simulink model "solid_ofc"  (R2020a)
settings: Solver=VariableStepAuto  StartTime=0.0  StopTime=simulation.stopTime  RelTol=1e-3
values from neighbouring files (symbols this model uses):
  MaxCrossings = 3    [solid_ofc_detection.m]
  Threshold = 0.1    [solid_ofc_detection.m]
  tp = 1/2/pi    (= 0.159154943092)    [solid_ofc_detection.m]
undefined symbols (not defined in the file or in its folder): simulation
libraries: simulink x1, dspsigops x1
settings Model: Creator=FawadFarooq  LastModifiedBy=FawaD KhaN
settings DebuggingCC: SFMachineParentedDataDiag=error

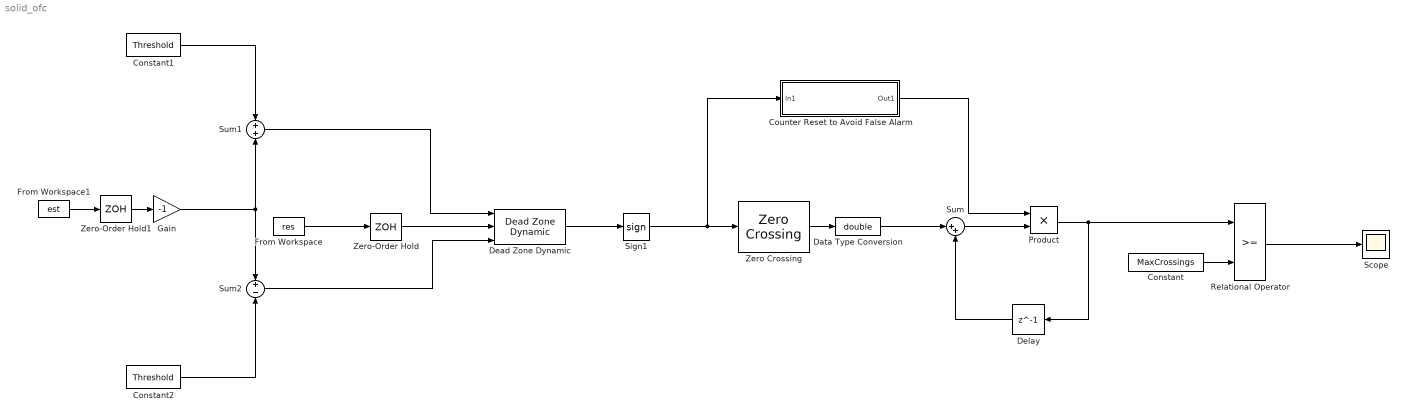
== system solid_ofc ==
  Constant : Constant  Value=MaxCrossings
  Constant1 : Constant  Value=Threshold
  Constant2 : Constant  Value=Threshold
  Counter Reset to Avoid False Alarm : Subsystem
  Data Type Conversion : DataTypeConversion  OutDataTypeStr=double
  Dead Zone Dynamic : simulink/Discontinuities/Dead Zone Dynamic
      settings: SourceProductBaseCode=SL
  Delay : Delay  DelayLength=1  SampleTime=1/simulation.Fs
  From Workspace : FromWorkspace  VariableName=res  SampleTime=1/simulation.Fs
  From Workspace1 : FromWorkspace  VariableName=est  SampleTime=1/simulation.Fs
  Gain : Gain  Gain=-1
  Product : Product
  Relational Operator : RelationalOperator  OutDataTypeStr=boolean  RndMeth=Simplest
  Scope : Scope
  Sign1 : Signum
  Sum : Sum  Inputs=|++
  Sum1 : Sum  Inputs=+|+
  Sum2 : Sum  Inputs=+|-
  Zero Crossing : dspsigops/Zero Crossing  InputProcessing=Columns as channels (frame based)
      settings: SourceProductBaseCode=DS
  Zero-Order Hold : ZeroOrderHold  SampleTime=1/simulation.Fs
  Zero-Order Hold1 : ZeroOrderHold  SampleTime=1/simulation.Fs
  wires:
  From Workspace/1 -> Zero-Order Hold/1
  Sign1/1 -> Counter Reset to Avoid False Alarm/1(In1), Zero Crossing/1
  Zero Crossing/1 -> Data Type Conversion/1
  Data Type Conversion/1 -> Sum/1
  Zero-Order Hold/1 -> Dead Zone Dynamic/2
  Delay/1 -> Sum/2
  Sum/1 -> Product/2
  Product/1 -> Delay/1, Relational Operator/1
  Constant/1 -> Relational Operator/2
  Relational Operator/1 -> Scope/1
  Counter Reset to Avoid False Alarm/1(Out1) -> Product/1
  From Workspace1/1 -> Zero-Order Hold1/1
  Zero-Order Hold1/1 -> Gain/1
  Constant1/1 -> Sum1/1
  Constant2/1 -> Sum2/2
  Sum2/1 -> Dead Zone Dynamic/3
  Sum1/1 -> Dead Zone Dynamic/1
  Gain/1 -> Sum1/2, Sum2/1
  Dead Zone Dynamic/1 -> Sign1/1

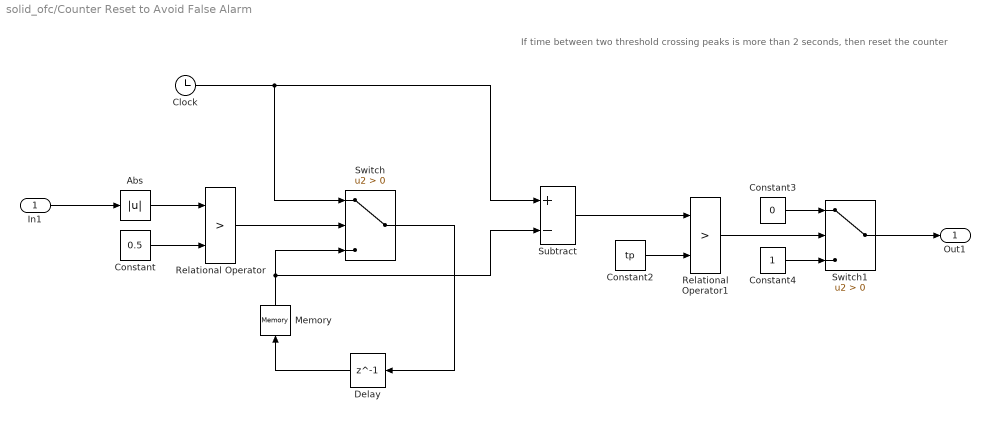
== system solid_ofc/Counter Reset to Avoid False Alarm ==
  note: If time between two threshold crossing peaks is more than 2 seconds, then reset the counter
  In1 : Inport
  Abs : Abs
  Clock : Clock
  Constant : Constant  Value=0.5
  Constant2 : Constant  Value=tp
  Constant3 : Constant  Value=0
  Constant4 : Constant
  Delay : Delay  DelayLength=1  SampleTime=1/simulation.Fs
  Memory : Memory
  Relational Operator : RelationalOperator  Operator=>  OutDataTypeStr=boolean  RndMeth=Simplest
  Relational Operator1 : RelationalOperator  Operator=>  OutDataTypeStr=boolean  RndMeth=Simplest
  Subtract : Sum  Inputs=+-
  Switch : Switch  Criteria=u2 > Threshold
  Switch1 : Switch  Criteria=u2 > Threshold
  Out1 : Outport
  wires:
  Switch1/1 -> Out1/1
  In1/1 -> Abs/1
  Abs/1 -> Relational Operator/1
  Constant/1 -> Relational Operator/2
  Relational Operator/1 -> Switch/2
  Switch/1 -> Delay/1
  Delay/1 -> Memory/1
  Memory/1 -> Subtract/2, Switch/3
  Clock/1 -> Subtract/1, Switch/1
  Subtract/1 -> Relational Operator1/1
  Constant2/1 -> Relational Operator1/2
  Relational Operator1/1 -> Switch1/2
  Constant3/1 -> Switch1/1
  Constant4/1 -> Switch1/3
